simulink model "simulator_with_observer"  (R2022a)
settings: Solver=VariableStepAuto  StartTime=0.0  StopTime=10  RelTol=1e-3  EnableMultiTasking=on
values from neighbouring files (symbols this model uses):
  A = [-1.4, 0.2, -0.1 ... (first row only)    [generate_simulations_model1.m]    (also in generate_simulations_model2.m = [-4.762, -634.92,   0)
  B1 = [1;1;1]    [generate_simulations_model1.m]    (also in generate_simulations_model2.m = [0 0 1]')
  B2 = [0.1, 0.8 ... (first row only)    [generate_simulations_model1.m]    (also in generate_simulations_model2.m = [0.4762, 0, 0]')
  bA = [A                 B1*Pi ... (first row only)    [generate_simulations_model1.m]    (also in generate_simulations_model2.m)
  bB2 = [B2; zeros((r+1)*q,m)]    [generate_simulations_model1.m]    (also in generate_simulations_model2.m)
  bC2 = [C D zeros(p,r*q)]    [generate_simulations_model1.m]    (also in generate_simulations_model2.m)
  C = eye(3)    [generate_simulations_model1.m]    (also in generate_simulations_model2.m)
  eta0 = [x0,b0+b1+b2,a0*w0+a1*w1+a2*w2,-b0*w0^2-b1*w1^2-b1*w1^2]    [generate_simulations_model1.m]    (also in generate_simulations_model2.m)
  Kw0 = -inv(R)*B2'*(-(A+B2*Kx)')^(-1)*S_T*B1    [generate_simulations_model1.m]    (also in generate_simulations_model2.m)
  Kw1 = -inv(R)*B2'*(-(A+B2*Kx)')^(-2)*S_T*B1    [generate_simulations_model1.m]    (also in generate_simulations_model2.m)
  Kw2 = -inv(R)*B2'*(-(A+B2*Kx)')^(-3)*S_T*B1    [generate_simulations_model1.m]    (also in generate_simulations_model2.m)
  Kx = -inv(R)*B2'*S_T    [generate_simulations_model1.m]    (also in generate_simulations_model2.m)
  L = place(bA', bC2', Obs_poles*[1.01 1.02 0.99 0.98 0.97 0.96])'    [generate_simulations_model1.m]    (also in generate_simulations_model2.m)
  m = 2    [generate_simulations_model1.m]    (also in generate_simulations_model2.m = 1)
  q = 1    [generate_simulations_model1.m]    (also in generate_simulations_model2.m)
  Q = eye(3)    [generate_simulations_model1.m]    (also in generate_simulations_model2.m)
  R = 0.1*eye(2)    [generate_simulations_model1.m]    (also in generate_simulations_model2.m = 0.1)
  x0 = [0, 0, 0]    [generate_simulations_model1.m]    (also in generate_simulations_model2.m)
settings Model: Creator=alcasfra  LastModifiedBy=CFV4mj
settings SolverCC: AlgebraicLoopSolver=TrustRegion
settings DataIOCC: ReturnWorkspaceOutputs=off
settings OptimizationCC: LifeSpan=inf
settings DebuggingCC: UnconnectedInputMsg=warning  UnconnectedOutputMsg=warning  UnconnectedLineMsg=warning  SFUnexpectedBacktrackingDiag=warning  SFNoUnconditionalDefaultTransitionDiag=warning  SFMachineParentedDataDiag=warning  ArithmeticOperatorsInVariantConditions=warning
settings SFSimCC: SimUseLocalCustomCode=off  CustomCodeUndefinedFunction=UseInterfaceOnly
settings RTWCC: RTWUseLocalCustomCode=off  DLArmComputeVersion=19.05
settings CodeAppCC: StateflowObjectComments=on
settings GRTTargetCC: TargetLangStandard=C89/C90 (ANSI)
settings ConfigComp: CovMetricSettings=dw  CovSaveCumulativeToWorkspaceVar=on  CovSaveSingleToWorkspaceVar=on  CovExternalEMLEnable=off

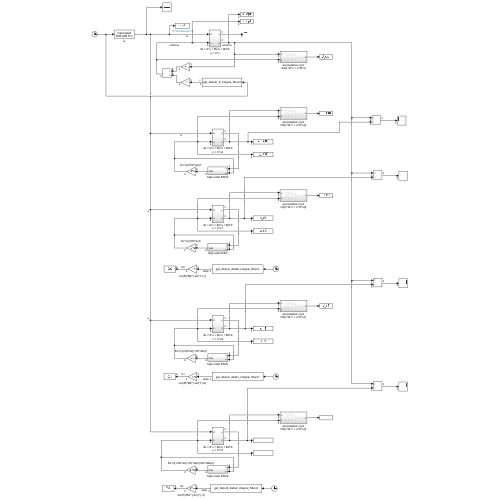
[thumbnail: Simulink's stored preview of the top-level diagram]
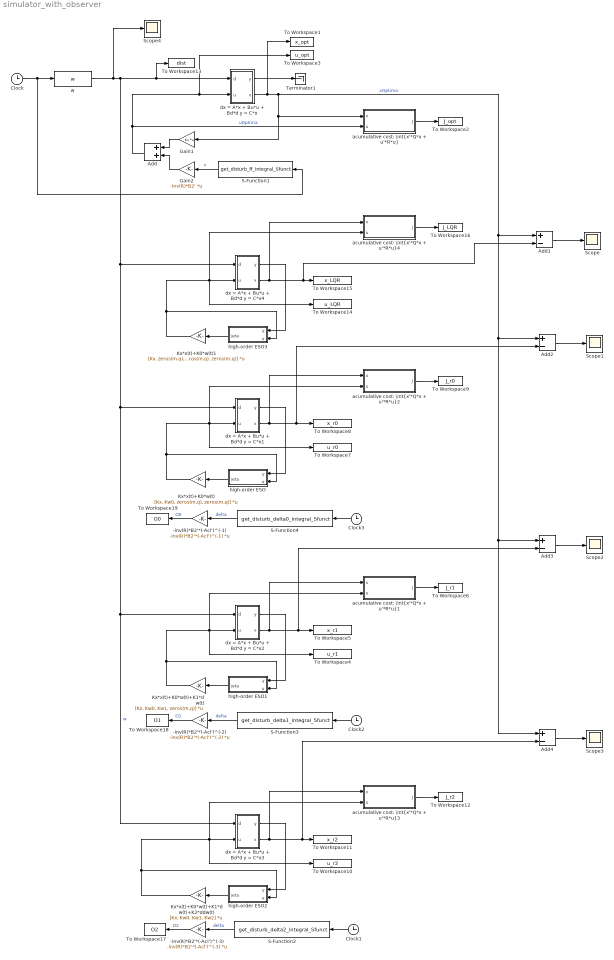
== system simulator_with_observer ==
  -inv(R)*B2'*(-Acl')^(-1) : Gain  Gain=-inv(R)*B2'*(-Acl')^(-1)  Multiplication=Matrix(K*u)
  -inv(R)*B2'*(-Acl')^(-2) : Gain  Gain=-inv(R)*B2'*(-Acl')^(-2)  Multiplication=Matrix(K*u)
  -inv(R)*B2'*(-Acl')^(-3) : Gain  Gain=-inv(R)*B2'*(-Acl')^(-3)  Multiplication=Matrix(K*u)
  Add : Sum
  Add{1..4} (4 alike) : Sum  Inputs=+-
  Clock{,1..3} (4 alike) : Clock
  Gain1 : Gain  Gain=Kx  Multiplication=Matrix(K*u)
  Gain2 : Gain  Gain=-inv(R)*B2'  Multiplication=Matrix(K*u)
  Kx*x(t)+K0*w(t) : Gain  Gain=[Kx, Kw0, zeros(m,q), zeros(m,q)]  Multiplication=Matrix(K*u)
  Kx*x(t)+K0*w(t)+K1*dw(t) : Gain  Gain=[Kx, Kw0, Kw1, zeros(m,q)]  Multiplication=Matrix(K*u)
  Kx*x(t)+K0*w(t)+K1*dw(t)+K2*ddw(t) : Gain  Gain=[Kx, Kw0, Kw1, Kw2]  Multiplication=Matrix(K*u)
  Kx*x(t)+K0*w(t)1 : Gain  Gain=[Kx, zeros(m,q), zeros(m,q), zeros(m,q)]  Multiplication=Matrix(K*u)
  S-Function1 : S-Function  FunctionName=get_disturb_ff_integral_Sfunct  Parameters=Acl, S_T, B1, h, delta  SFunctionDeploymentMode=off  EnableBusSupport=off
  S-Function2 : S-Function  FunctionName=get_disturb_delta2_integral_Sfunct  Parameters=Acl, S_T, B1, h, delta  SFunctionDeploymentMode=off  EnableBusSupport=off
  S-Function3 : S-Function  FunctionName=get_disturb_delta1_integral_Sfunct  Parameters=Acl, S_T, B1, h, delta  SFunctionDeploymentMode=off  EnableBusSupport=off
  S-Function4 : S-Function  FunctionName=get_disturb_delta0_integral_Sfunct  Parameters=Acl, S_T, B1, h, delta  SFunctionDeploymentMode=off  EnableBusSupport=off
  Scope{,1..4} (5 alike) : Scope
  Terminator1 : Terminator
  To Workspace1 : ToWorkspace  VariableName=x_opt  SaveFormat=Structure With Time  SampleTime=-1
  To Workspace10 : ToWorkspace  VariableName=u_r2  SaveFormat=Structure With Time  SampleTime=-1
  To Workspace11 : ToWorkspace  VariableName=x_r2  SaveFormat=Structure With Time  SampleTime=-1
  To Workspace12 : ToWorkspace  VariableName=J_r2  SaveFormat=Structure With Time  SampleTime=-1
  To Workspace13 : ToWorkspace  VariableName=dist  SaveFormat=Structure With Time  SampleTime=-1
  To Workspace14 : ToWorkspace  VariableName=u_LQR  SaveFormat=Structure With Time  SampleTime=-1
  To Workspace15 : ToWorkspace  VariableName=x_LQR  SaveFormat=Structure With Time  SampleTime=-1
  To Workspace16 : ToWorkspace  VariableName=J_LQR  SaveFormat=Structure With Time  SampleTime=-1
  To Workspace17 : ToWorkspace  VariableName=O2  SaveFormat=Structure With Time  SampleTime=-1
  To Workspace18 : ToWorkspace  VariableName=O1  SaveFormat=Structure With Time  SampleTime=-1
  To Workspace19 : ToWorkspace  VariableName=O0  SaveFormat=Structure With Time  SampleTime=-1
  To Workspace2 : ToWorkspace  VariableName=J_opt  SaveFormat=Structure With Time  SampleTime=-1
  To Workspace3 : ToWorkspace  VariableName=u_opt  SaveFormat=Structure With Time  SampleTime=-1
  To Workspace4 : ToWorkspace  VariableName=u_r1  SaveFormat=Structure With Time  SampleTime=-1
  To Workspace5 : ToWorkspace  VariableName=x_r1  SaveFormat=Structure With Time  SampleTime=-1
  To Workspace6 : ToWorkspace  VariableName=J_r1  SaveFormat=Structure With Time  SampleTime=-1
  To Workspace7 : ToWorkspace  VariableName=u_r0  SaveFormat=Structure With Time  SampleTime=-1
  To Workspace8 : ToWorkspace  VariableName=x_r0  SaveFormat=Structure With Time  SampleTime=-1
  To Workspace9 : ToWorkspace  VariableName=J_r0  SaveFormat=Structure With Time  SampleTime=-1
  "acumulative cost: \\int{x'*Q*x + u'*R*u}" : Subsystem
  "acumulative cost: \\int{x'*Q*x + u'*R*u}1" : Subsystem
  "acumulative cost: \\int{x'*Q*x + u'*R*u}2" : Subsystem
  "acumulative cost: \\int{x'*Q*x + u'*R*u}3" : Subsystem
  "acumulative cost: \\int{x'*Q*x + u'*R*u}4" : Subsystem
  dx = A*x + Bu*u + Bd*d y = C*x : Subsystem
  dx = A*x + Bu*u + Bd*d y = C*x1 : Subsystem
  dx = A*x + Bu*u + Bd*d y = C*x2 : Subsystem
  dx = A*x + Bu*u + Bd*d y = C*x3 : Subsystem
  dx = A*x + Bu*u + Bd*d y = C*x4 : Subsystem
  high-order ESO : Subsystem
  high-order ESO1 : Subsystem
  high-order ESO2 : Subsystem
  high-order ESO3 : Subsystem
  w : MATLABFcn  MATLABFcn=w
  wires:
  Add/1 -> "acumulative cost: \\int{x'*Q*x + u'*R*u}"/2(u), To Workspace3/1, dx = A*x + Bu*u + Bd*d y = C*x/2(u)  "uOptima"
  dx = A*x + Bu*u + Bd*d y = C*x/2(x) -> To Workspace1/1, Add4/1, Add3/1, Add2/1, Add1/1, Gain1/1, "acumulative cost: \\int{x'*Q*x + u'*R*u}"/1(x)  "xOptimo"
  Gain1/1 -> Add/1
  dx = A*x + Bu*u + Bd*d y = C*x/1(y) -> Terminator1/1
  "acumulative cost: \\int{x'*Q*x + u'*R*u}"/1(J) -> To Workspace2/1
  S-Function1/1 -> Gain2/1  "v"
  Gain2/1 -> Add/2
  dx = A*x + Bu*u + Bd*d y = C*x1/1(y) -> high-order ESO/1(y)
  high-order ESO/1(\eta) -> Kx*x(t)+K0*w(t)/1
  Kx*x(t)+K0*w(t)/1 -> high-order ESO/2(u), To Workspace7/1, "acumulative cost: \\int{x'*Q*x + u'*R*u}2"/2(u), dx = A*x + Bu*u + Bd*d y = C*x1/2(u)
  "acumulative cost: \\int{x'*Q*x + u'*R*u}2"/1(J) -> To Workspace9/1
  dx = A*x + Bu*u + Bd*d y = C*x1/2(x) -> Add2/2, To Workspace8/1, "acumulative cost: \\int{x'*Q*x + u'*R*u}2"/1(x)
  dx = A*x + Bu*u + Bd*d y = C*x2/2(x) -> Add3/2, To Workspace5/1, "acumulative cost: \\int{x'*Q*x + u'*R*u}1"/1(x)
  "acumulative cost: \\int{x'*Q*x + u'*R*u}1"/1(J) -> To Workspace6/1
  Kx*x(t)+K0*w(t)+K1*dw(t)/1 -> high-order ESO1/2(u), To Workspace4/1, "acumulative cost: \\int{x'*Q*x + u'*R*u}1"/2(u), dx = A*x + Bu*u + Bd*d y = C*x2/2(u)
  dx = A*x + Bu*u + Bd*d y = C*x2/1(y) -> high-order ESO1/1(y)
  dx = A*x + Bu*u + Bd*d y = C*x3/1(y) -> high-order ESO2/1(y)
  "acumulative cost: \\int{x'*Q*x + u'*R*u}3"/1(J) -> To Workspace12/1
  Clock/1 -> S-Function1/1, w/1
  Kx*x(t)+K0*w(t)1/1 -> high-order ESO3/2(u), To Workspace14/1, "acumulative cost: \\int{x'*Q*x + u'*R*u}4"/2(u), dx = A*x + Bu*u + Bd*d y = C*x4/2(u)
  "acumulative cost: \\int{x'*Q*x + u'*R*u}4"/1(J) -> To Workspace16/1
  dx = A*x + Bu*u + Bd*d y = C*x4/1(y) -> high-order ESO3/1(y)
  w/1 -> Scope4/1, dx = A*x + Bu*u + Bd*d y = C*x3/1(d), dx = A*x + Bu*u + Bd*d y = C*x2/1(d), dx = A*x + Bu*u + Bd*d y = C*x1/1(d), dx = A*x + Bu*u + Bd*d y = C*x4/1(d), To Workspace13/1, dx = A*x + Bu*u + Bd*d y = C*x/1(d)  "w"
  high-order ESO3/1(\eta) -> Kx*x(t)+K0*w(t)1/1
  dx = A*x + Bu*u + Bd*d y = C*x4/2(x) -> Add1/2, To Workspace15/1, "acumulative cost: \\int{x'*Q*x + u'*R*u}4"/1(x)
  dx = A*x + Bu*u + Bd*d y = C*x3/2(x) -> Add4/2, To Workspace11/1, "acumulative cost: \\int{x'*Q*x + u'*R*u}3"/1(x)
  high-order ESO2/1(\eta) -> Kx*x(t)+K0*w(t)+K1*dw(t)+K2*ddw(t)/1
  high-order ESO1/1(\eta) -> Kx*x(t)+K0*w(t)+K1*dw(t)/1
  Clock1/1 -> S-Function2/1
  S-Function2/1 -> -inv(R)*B2'*(-Acl')^(-3)/1  "delta"
  -inv(R)*B2'*(-Acl')^(-3)/1 -> To Workspace17/1  "O2"
  Kx*x(t)+K0*w(t)+K1*dw(t)+K2*ddw(t)/1 -> high-order ESO2/2(u), To Workspace10/1, "acumulative cost: \\int{x'*Q*x + u'*R*u}3"/2(u), dx = A*x + Bu*u + Bd*d y = C*x3/2(u)
  Clock2/1 -> S-Function3/1
  S-Function3/1 -> -inv(R)*B2'*(-Acl')^(-2)/1  "delta"
  -inv(R)*B2'*(-Acl')^(-2)/1 -> To Workspace18/1  "O1"
  -inv(R)*B2'*(-Acl')^(-1)/1 -> To Workspace19/1  "O0"
  S-Function4/1 -> -inv(R)*B2'*(-Acl')^(-1)/1  "delta"
  Clock3/1 -> S-Function4/1
  Add1/1 -> Scope/1
  Add2/1 -> Scope1/1
  Add3/1 -> Scope2/1
  Add4/1 -> Scope3/1

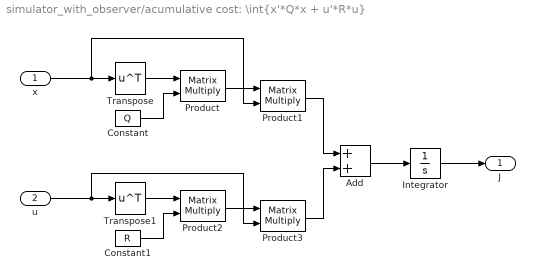
== system simulator_with_observer/acumulative cost: \int{x'*Q*x + u'*R*u} ==
  x : Inport
  u : Inport  Port=2
  Add : Sum
  Constant : Constant  Value=Q
  Constant1 : Constant  Value=R
  Integrator : Integrator
  Product{,1..3} (4 alike) : Product  Multiplication=Matrix(*)
  Transpose : Math  Operator=transpose  SignedPower=on
  Transpose1 : Math  Operator=transpose  SignedPower=on
  J : Outport  VectorParamsAs1DForOutWhenUnconnected=off
  wires:
  Add/1 -> Integrator/1
  Constant/1 -> Product/2
  Product/1 -> Product1/1
  x/1 -> Product1/2, Transpose/1
  Integrator/1 -> J/1
  Transpose/1 -> Product/1
  Transpose1/1 -> Product2/1
  Product2/1 -> Product3/1
  Constant1/1 -> Product2/2
  u/1 -> Transpose1/1, Product3/2
  Product1/1 -> Add/1
  Product3/1 -> Add/2

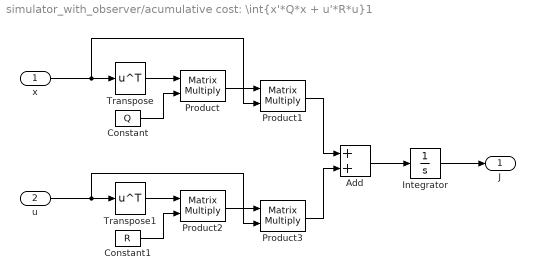
== system simulator_with_observer/acumulative cost: \int{x'*Q*x + u'*R*u}1 ==
  x : Inport
  u : Inport  Port=2
  Add : Sum
  Constant : Constant  Value=Q
  Constant1 : Constant  Value=R
  Integrator : Integrator
  Product{,1..3} (4 alike) : Product  Multiplication=Matrix(*)
  Transpose : Math  Operator=transpose  SignedPower=on
  Transpose1 : Math  Operator=transpose  SignedPower=on
  J : Outport  VectorParamsAs1DForOutWhenUnconnected=off
  wires:
  Product3/1 -> Add/2
  Product1/1 -> Add/1
  u/1 -> Product3/2, Transpose1/1
  Constant1/1 -> Product2/2
  Product2/1 -> Product3/1
  Transpose1/1 -> Product2/1
  Transpose/1 -> Product/1
  Integrator/1 -> J/1
  x/1 -> Transpose/1, Product1/2
  Product/1 -> Product1/1
  Constant/1 -> Product/2
  Add/1 -> Integrator/1

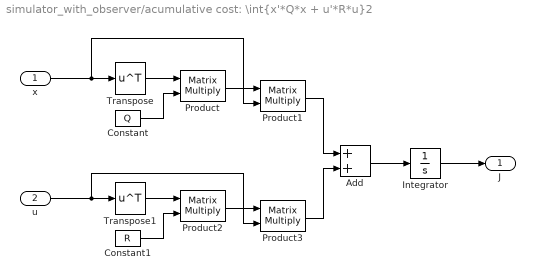
== system simulator_with_observer/acumulative cost: \int{x'*Q*x + u'*R*u}2 ==
  x : Inport
  u : Inport  Port=2
  Add : Sum
  Constant : Constant  Value=Q
  Constant1 : Constant  Value=R
  Integrator : Integrator
  Product{,1..3} (4 alike) : Product  Multiplication=Matrix(*)
  Transpose : Math  Operator=transpose  SignedPower=on
  Transpose1 : Math  Operator=transpose  SignedPower=on
  J : Outport  VectorParamsAs1DForOutWhenUnconnected=off
  wires:
  Product3/1 -> Add/2
  Product1/1 -> Add/1
  u/1 -> Product3/2, Transpose1/1
  Constant1/1 -> Product2/2
  Product2/1 -> Product3/1
  Transpose1/1 -> Product2/1
  Transpose/1 -> Product/1
  Integrator/1 -> J/1
  x/1 -> Transpose/1, Product1/2
  Product/1 -> Product1/1
  Constant/1 -> Product/2
  Add/1 -> Integrator/1

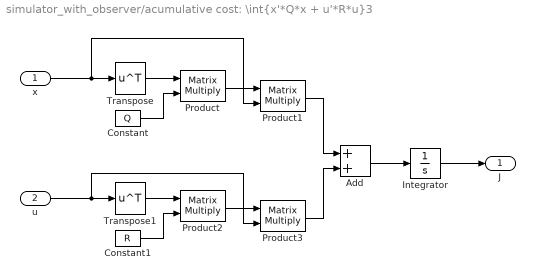
== system simulator_with_observer/acumulative cost: \int{x'*Q*x + u'*R*u}3 ==
  x : Inport
  u : Inport  Port=2
  Add : Sum
  Constant : Constant  Value=Q
  Constant1 : Constant  Value=R
  Integrator : Integrator
  Product{,1..3} (4 alike) : Product  Multiplication=Matrix(*)
  Transpose : Math  Operator=transpose  SignedPower=on
  Transpose1 : Math  Operator=transpose  SignedPower=on
  J : Outport  VectorParamsAs1DForOutWhenUnconnected=off
  wires:
  Product3/1 -> Add/2
  Product1/1 -> Add/1
  u/1 -> Product3/2, Transpose1/1
  Constant1/1 -> Product2/2
  Product2/1 -> Product3/1
  Transpose1/1 -> Product2/1
  Transpose/1 -> Product/1
  Integrator/1 -> J/1
  x/1 -> Transpose/1, Product1/2
  Product/1 -> Product1/1
  Constant/1 -> Product/2
  Add/1 -> Integrator/1

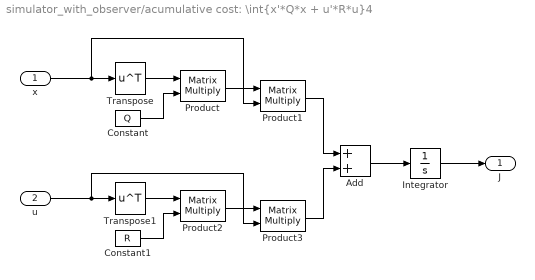
== system simulator_with_observer/acumulative cost: \int{x'*Q*x + u'*R*u}4 ==
  x : Inport
  u : Inport  Port=2
  Add : Sum
  Constant : Constant  Value=Q
  Constant1 : Constant  Value=R
  Integrator : Integrator
  Product{,1..3} (4 alike) : Product  Multiplication=Matrix(*)
  Transpose : Math  Operator=transpose  SignedPower=on
  Transpose1 : Math  Operator=transpose  SignedPower=on
  J : Outport  VectorParamsAs1DForOutWhenUnconnected=off
  wires:
  Product3/1 -> Add/2
  Product1/1 -> Add/1
  u/1 -> Product3/2, Transpose1/1
  Constant1/1 -> Product2/2
  Product2/1 -> Product3/1
  Transpose1/1 -> Product2/1
  Transpose/1 -> Product/1
  Integrator/1 -> J/1
  x/1 -> Transpose/1, Product1/2
  Product/1 -> Product1/1
  Constant/1 -> Product/2
  Add/1 -> Integrator/1

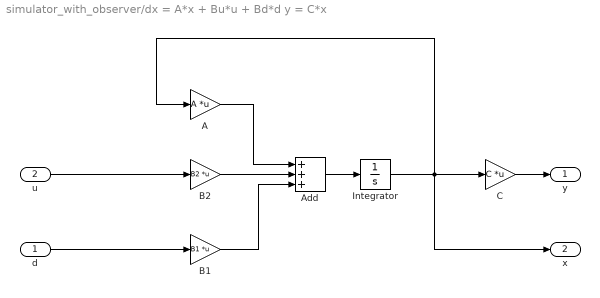
== system simulator_with_observer/dx = A*x + Bu*u + Bd*d y = C*x ==
  d : Inport
  u : Inport  Port=2
  A : Gain  Gain=A  Multiplication=Matrix(K*u)
  Add : Sum  Inputs=+++
  B1 : Gain  Gain=B1  Multiplication=Matrix(K*u)
  B2 : Gain  Gain=B2  Multiplication=Matrix(K*u)
  C : Gain  Gain=C  Multiplication=Matrix(K*u)
  Integrator : Integrator  InitialCondition=x0
  y : Outport  VectorParamsAs1DForOutWhenUnconnected=off
  x : Outport  Port=2  VectorParamsAs1DForOutWhenUnconnected=off
  wires:
  Integrator/1 -> A/1, C/1, x/1
  C/1 -> y/1
  A/1 -> Add/1
  u/1 -> B2/1
  Add/1 -> Integrator/1
  B2/1 -> Add/2
  B1/1 -> Add/3
  d/1 -> B1/1

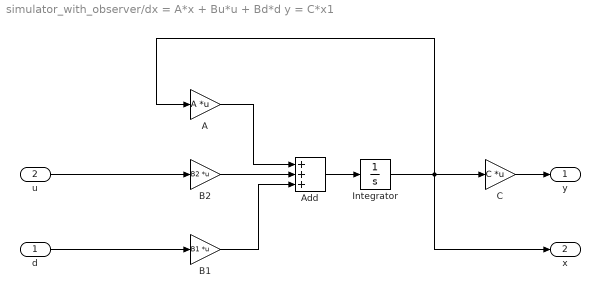
== system simulator_with_observer/dx = A*x + Bu*u + Bd*d y = C*x1 ==
  d : Inport
  u : Inport  Port=2
  A : Gain  Gain=A  Multiplication=Matrix(K*u)
  Add : Sum  Inputs=+++
  B1 : Gain  Gain=B1  Multiplication=Matrix(K*u)
  B2 : Gain  Gain=B2  Multiplication=Matrix(K*u)
  C : Gain  Gain=C  Multiplication=Matrix(K*u)
  Integrator : Integrator  InitialCondition=x0
  y : Outport  VectorParamsAs1DForOutWhenUnconnected=off
  x : Outport  Port=2  VectorParamsAs1DForOutWhenUnconnected=off
  wires:
  d/1 -> B1/1
  B1/1 -> Add/3
  B2/1 -> Add/2
  Add/1 -> Integrator/1
  u/1 -> B2/1
  A/1 -> Add/1
  C/1 -> y/1
  Integrator/1 -> x/1, C/1, A/1

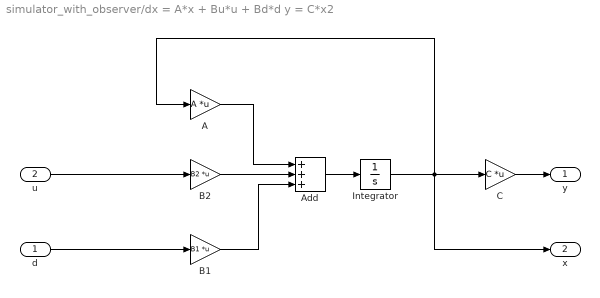
== system simulator_with_observer/dx = A*x + Bu*u + Bd*d y = C*x2 ==
  d : Inport
  u : Inport  Port=2
  A : Gain  Gain=A  Multiplication=Matrix(K*u)
  Add : Sum  Inputs=+++
  B1 : Gain  Gain=B1  Multiplication=Matrix(K*u)
  B2 : Gain  Gain=B2  Multiplication=Matrix(K*u)
  C : Gain  Gain=C  Multiplication=Matrix(K*u)
  Integrator : Integrator  InitialCondition=x0
  y : Outport  VectorParamsAs1DForOutWhenUnconnected=off
  x : Outport  Port=2  VectorParamsAs1DForOutWhenUnconnected=off
  wires:
  d/1 -> B1/1
  B1/1 -> Add/3
  B2/1 -> Add/2
  Add/1 -> Integrator/1
  u/1 -> B2/1
  A/1 -> Add/1
  C/1 -> y/1
  Integrator/1 -> x/1, C/1, A/1

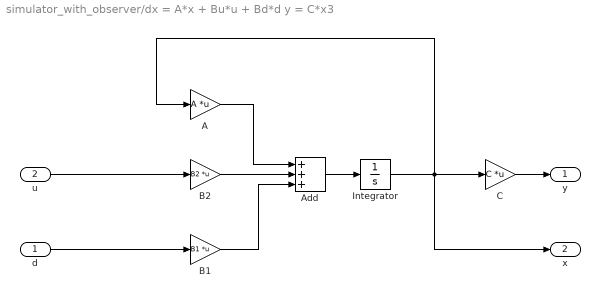
== system simulator_with_observer/dx = A*x + Bu*u + Bd*d y = C*x3 ==
  d : Inport
  u : Inport  Port=2
  A : Gain  Gain=A  Multiplication=Matrix(K*u)
  Add : Sum  Inputs=+++
  B1 : Gain  Gain=B1  Multiplication=Matrix(K*u)
  B2 : Gain  Gain=B2  Multiplication=Matrix(K*u)
  C : Gain  Gain=C  Multiplication=Matrix(K*u)
  Integrator : Integrator  InitialCondition=x0
  y : Outport  VectorParamsAs1DForOutWhenUnconnected=off
  x : Outport  Port=2  VectorParamsAs1DForOutWhenUnconnected=off
  wires:
  d/1 -> B1/1
  B1/1 -> Add/3
  B2/1 -> Add/2
  Add/1 -> Integrator/1
  u/1 -> B2/1
  A/1 -> Add/1
  C/1 -> y/1
  Integrator/1 -> x/1, C/1, A/1

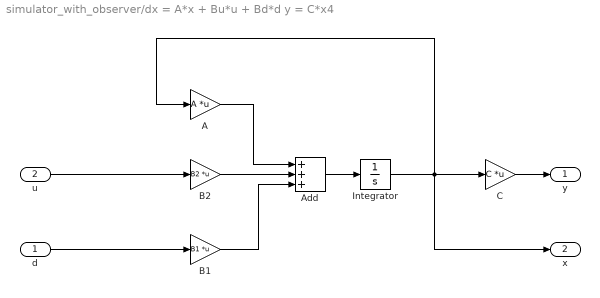
== system simulator_with_observer/dx = A*x + Bu*u + Bd*d y = C*x4 ==
  d : Inport
  u : Inport  Port=2
  A : Gain  Gain=A  Multiplication=Matrix(K*u)
  Add : Sum  Inputs=+++
  B1 : Gain  Gain=B1  Multiplication=Matrix(K*u)
  B2 : Gain  Gain=B2  Multiplication=Matrix(K*u)
  C : Gain  Gain=C  Multiplication=Matrix(K*u)
  Integrator : Integrator  InitialCondition=x0
  y : Outport  VectorParamsAs1DForOutWhenUnconnected=off
  x : Outport  Port=2  VectorParamsAs1DForOutWhenUnconnected=off
  wires:
  d/1 -> B1/1
  B1/1 -> Add/3
  B2/1 -> Add/2
  Add/1 -> Integrator/1
  u/1 -> B2/1
  A/1 -> Add/1
  C/1 -> y/1
  Integrator/1 -> x/1, C/1, A/1

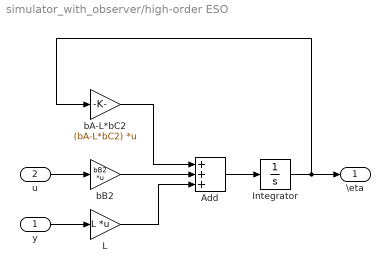
== system simulator_with_observer/high-order ESO ==
  y : Inport
  u : Inport  Port=2
  Add : Sum  Inputs=+++
  Integrator : Integrator  InitialCondition=eta0
  L : Gain  Gain=L  Multiplication=Matrix(K*u)
  bA-L*bC2 : Gain  Gain=(bA-L*bC2)  Multiplication=Matrix(K*u)
  bB2 : Gain  Gain=bB2  Multiplication=Matrix(K*u)
  \eta : Outport  VectorParamsAs1DForOutWhenUnconnected=off
  wires:
  y/1 -> L/1
  L/1 -> Add/3
  bB2/1 -> Add/2
  Add/1 -> Integrator/1
  u/1 -> bB2/1
  bA-L*bC2/1 -> Add/1
  Integrator/1 -> bA-L*bC2/1, \eta/1

== system simulator_with_observer/high-order ESO1 ==
  y : Inport
  u : Inport  Port=2
  Add : Sum  Inputs=+++
  Integrator : Integrator  InitialCondition=eta0
  L : Gain  Gain=L  Multiplication=Matrix(K*u)
  bA-L*bC2 : Gain  Gain=(bA-L*bC2)  Multiplication=Matrix(K*u)
  bB2 : Gain  Gain=bB2  Multiplication=Matrix(K*u)
  \eta : Outport  VectorParamsAs1DForOutWhenUnconnected=off
  wires:
  y/1 -> L/1
  L/1 -> Add/3
  bB2/1 -> Add/2
  Add/1 -> Integrator/1
  u/1 -> bB2/1
  bA-L*bC2/1 -> Add/1
  Integrator/1 -> bA-L*bC2/1, \eta/1

== system simulator_with_observer/high-order ESO2 ==
  y : Inport
  u : Inport  Port=2
  Add : Sum  Inputs=+++
  Integrator : Integrator  InitialCondition=eta0
  L : Gain  Gain=L  Multiplication=Matrix(K*u)
  bA-L*bC2 : Gain  Gain=(bA-L*bC2)  Multiplication=Matrix(K*u)
  bB2 : Gain  Gain=bB2  Multiplication=Matrix(K*u)
  \eta : Outport  VectorParamsAs1DForOutWhenUnconnected=off
  wires:
  y/1 -> L/1
  L/1 -> Add/3
  bB2/1 -> Add/2
  Add/1 -> Integrator/1
  u/1 -> bB2/1
  bA-L*bC2/1 -> Add/1
  Integrator/1 -> bA-L*bC2/1, \eta/1

== system simulator_with_observer/high-order ESO3 ==
  y : Inport
  u : Inport  Port=2
  Add : Sum  Inputs=+++
  Integrator : Integrator  InitialCondition=eta0
  L : Gain  Gain=L  Multiplication=Matrix(K*u)
  bA-L*bC2 : Gain  Gain=(bA-L*bC2)  Multiplication=Matrix(K*u)
  bB2 : Gain  Gain=bB2  Multiplication=Matrix(K*u)
  \eta : Outport  VectorParamsAs1DForOutWhenUnconnected=off
  wires:
  y/1 -> L/1
  L/1 -> Add/3
  bB2/1 -> Add/2
  Add/1 -> Integrator/1
  u/1 -> bB2/1
  bA-L*bC2/1 -> Add/1
  Integrator/1 -> bA-L*bC2/1, \eta/1
